simulink model "TTypeInverter_R2022a"  (R2022a)
settings: Solver=ode23t  StartTime=0.0  StopTime=0.2  RelTol=1e-3  EnableMultiTasking=on
values from neighbouring files (symbols this model uses):
  C_c = 30*10^-6    (= 3e-05)    [TTypeInverterVals.m]
  den = abs(G_pr_r_z.Denominator{1,1})    [TTypeInverterVals.m]
  den15 = abs(G_pr_r_15_z.Denominator{1,1})    [TTypeInverterVals.m]
  den21 = abs(G_pr_r_21_z.Denominator{1,1})    [TTypeInverterVals.m]
  den5 = abs(G_pr_r_5_z.Denominator{1,1})    [TTypeInverterVals.m]
  den7 = abs(G_pr_r_7_z.Denominator{1,1})    [TTypeInverterVals.m]
  f_o = 50    [TTypeInverterVals.m]
  G_diff_z = c2d(G_diff_s,Ts,opt)    [ControllerDesign.m]    (also in TTypeInverterVals.m = c2d(G_diff_s,Ts,'foh'))
  Kc = 2.5    [ControllerDesign.m]    (also in TTypeInverterVals.m)
  Klim = 5    [TTypeInverterVals.m]
  Kp = 1/mag/(10^(1.14/20))    [ControllerDesign.m]    (also in TTypeInverterVals.m = 0.9444)
  Kr = omega_c_o/2    (= 3141.59265359)    [ControllerDesign.m]    (also in TTypeInverterVals.m)
  N = 26    [Inductance.m]    (also in TTypeInverterVals.m = [0])
  num = abs(G_pr_r_z.Numerator{1,1})    [TTypeInverterVals.m]
  num15 = abs(G_pr_r_15_z.Numerator{1,1})    [TTypeInverterVals.m]
  num21 = abs(G_pr_r_21_z.Numerator{1,1})    [TTypeInverterVals.m]
  num5 = abs(G_pr_r_5_z.Numerator{1,1})    [TTypeInverterVals.m]
  num7 = abs(G_pr_r_7_z.Numerator{1,1})    [TTypeInverterVals.m]
  omega_o = fo*2*pi    (= 314.159265359)    [ControllerDesign.m]    (also in TTypeInverterVals.m)
  omega_w = 0.1*2*pi    (= 0.628318530718)    [ControllerDesign.m]    (also in TTypeInverterVals.m)
  pr_sat_val = ceil(3*io_nom)    [TTypeInverterVals.m]
  Q = eye(3)    [TTypeInverterVals.m]
  R = [R_iL 0 ... (first row only)    [TTypeInverterVals.m]
  R_l_20p = Vout^2/P_lin_20p    (= 10.58)    [TTypeInverterVals.m]
  R_l_3p = Vout/(P_max_3p/(Vout*3))    (= 2.116)    [TTypeInverterVals.m]
  R_l_80p = Vout^2/P_lin_80p    (= 2.645)    [TTypeInverterVals.m]
  R_l_nl = Vout^2/P_lin    (= 3.11176470588)    [TTypeInverterVals.m]
  R_l_nl_3p = Vout_3p^2/P_lin_3p    [TTypeInverterVals.m]
  R_Lc = 5.6e-3    (= 0.0056)    [TTypeInverterVals.m]
  R_nl_load = Uc^2/(0.66*S_tot)    (= 14.9121893939)    [TTypeInverterVals.m]
  R_nl_load_3p = Uc_3p^2/(0.66*S_tot_3p)    (= 4.97072979798)    [TTypeInverterVals.m]
  R_nl_s = 0.04*Vout^2/S_tot    (= 0.2645)    [TTypeInverterVals.m]
  R_nl_s_3p = 0.04*Vout_3p^2/S_tot_3p    [TTypeInverterVals.m]
  T_sw = 1/f_sw    (= 4.16666666667e-05)    [TTypeInverterVals.m]
  Tcomp = Ts/4    (= 2.60400009204e-06)    [TTypeInverterVals.m]
  Ts = 1/fs    (= 1.04166666667e-05)    [ControllerDesign.m]    (also in KalmanFilter.m = 2.08333333333e-05; TTypeInverterVals.m = 1.04160003681e-05)
  VDC = 800    [TTypeInverterVals.m]
  Vout_amp = Vout*sqrt(2)    [TTypeInverterVals.m]
undefined symbols (not defined in the file or in its folder): a0, a1, b0, b1, Discrete, G_ll_z, Ki, Kpc, KT, kv, Time, UKF_data
libraries: ee_lib x94, nesl_utility x48, fl_lib x39, dspstat3 x15, spsTriangleGeneratorLib x6, ctrlSharedLib x3, spsRMSLib x3, spsTHDLib x3
(part 4 of 5)

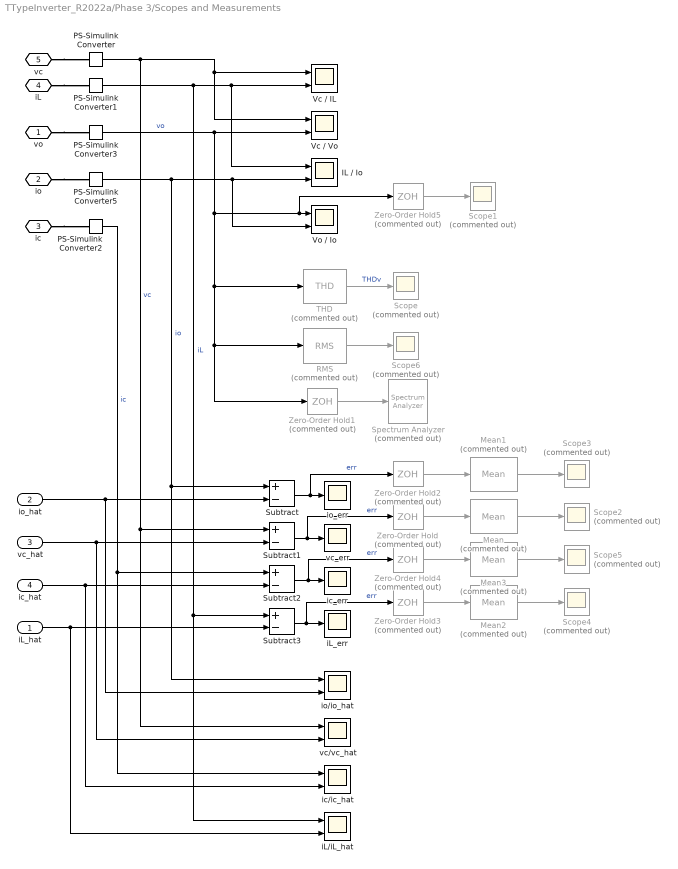
== system TTypeInverter_R2022a/Phase 3/Scopes and Measurements ==
  iL_hat : Inport
  io_hat : Inport  Port=2
  vc_hat : Inport  Port=3
  ic_hat : Inport  Port=4
  IL / Io : Scope  NumInputPorts=2
  Mean{,1..3} (4 alike) : dspstat3/Mean  Commented=on  run=on  InputProcessing=Columns as channels (frame based)  reset_popup=None  directionMode=Each column  dimension=1  roiEnable=off  roiType=Rectangles  roiPortion=Entire ROI  roiOutput=Individual statistics for each ROI  roiFlag=off  roundingMode=Floor  overflowMode=off  outputDataTypeStr=Inherit: Same as accumulator  outputMin=[]  outputMax=[]  outputLastDataTypeStr=Inherit: Same as accumulator
  PS-Simulink Converter{,1..3,5} (5 alike) : nesl_utility/PS-Simulink Converter  PhysicalDomain=network_engine_domain  SubClassName=ps_output  LeftPortType=input  RightPortType=output  PseudoPeriodic=off  Frequencies=[]  VectorFormat=inherit  Unit=inherit  AffineConversion=off
      settings: SourceProductBaseCode=SS,PW,VE
  RMS : spsRMSLib/RMS  Commented=on  TrueRMS=on  Freq=100  RMSInit=230  Ts=0
  Scope{,1..6} (7 alike) : Scope  Commented=on
  Spectrum Analyzer : SpectrumAnalyzer  Commented=on
  Subtract{,1..3} (4 alike) : Sum  Inputs=+-
  THD : spsTHDLib/THD  Commented=on  Freq=50  Ts=0
      settings: SourceProductBaseCode=PS
  Vc / IL : Scope  NumInputPorts=2
  Vc / Vo : Scope  NumInputPorts=2
  Vo / Io : Scope  NumInputPorts=2
  Zero-Order Hold{,2..4} (4 alike) : ZeroOrderHold  Commented=on  SampleTime=Ts/10
  Zero-Order Hold1 : ZeroOrderHold  Commented=on  SampleTime=1/100000
  Zero-Order Hold5 : ZeroOrderHold  Commented=on  SampleTime=T_sw/500
  iL/iL_hat : Scope  NumInputPorts=2
  iL_err : Scope
  ic/ic_hat : Scope  NumInputPorts=2
  ic_err : Scope
  io/io_hat : Scope  NumInputPorts=2
  io_err : Scope
  vc/vc_hat : Scope  NumInputPorts=2
  vc_err : Scope
  vo : PMIOPort  Side=Left
  io : PMIOPort  Port=2  Side=Left
  ic : PMIOPort  Port=3  Side=Left
  iL : PMIOPort  Port=4  Side=Left
  vc : PMIOPort  Port=5  Side=Left
  wires:
  PS-Simulink Converter1/1 -> iL/iL_hat/1, Subtract3/1, IL / Io/1, Vc / IL/2  "iL"
  PS-Simulink Converter/1 -> vc/vc_hat/1, Subtract1/1, Vc / Vo/1, Vc / IL/1  "vc"
  THD/1 -> Scope/1  "THDv"
  PS-Simulink Converter5/1 -> io/io_hat/1, Subtract/1, Vo / Io/2, IL / Io/2  "io"
  Zero-Order Hold1/1 -> Spectrum Analyzer/1
  io_hat/1 -> io/io_hat/2, Subtract/2
  Subtract/1 -> Zero-Order Hold2/1, io_err/1  "err"
  ic_hat/1 -> ic/ic_hat/2, Subtract2/2
  vc_hat/1 -> vc/vc_hat/2, Subtract1/2
  Subtract1/1 -> Zero-Order Hold/1, vc_err/1  "err"
  PS-Simulink Converter2/1 -> ic/ic_hat/1, Subtract2/1  "ic"
  Subtract2/1 -> Zero-Order Hold4/1, ic_err/1  "err"
  Mean/1 -> Scope2/1
  Zero-Order Hold/1 -> Mean/1
  Mean1/1 -> Scope3/1
  Zero-Order Hold2/1 -> Mean1/1
  iL_hat/1 -> iL/iL_hat/2, Subtract3/2
  Subtract3/1 -> Zero-Order Hold3/1, iL_err/1  "err"
  Mean2/1 -> Scope4/1
  Zero-Order Hold3/1 -> Mean2/1
  Mean3/1 -> Scope5/1
  Zero-Order Hold4/1 -> Mean3/1
  RMS/1 -> Scope6/1
  PS-Simulink Converter3/1 -> Vc / Vo/2, Zero-Order Hold5/1, Vo / Io/1, THD/1, RMS/1, Zero-Order Hold1/1  "vo"
  Zero-Order Hold5/1 -> Scope1/1
  connections:
  vc/RConn1 -- PS-Simulink Converter/LConn1
  iL/RConn1 -- PS-Simulink Converter1/LConn1
  vo/RConn1 -- PS-Simulink Converter3/LConn1
  io/RConn1 -- PS-Simulink Converter5/LConn1
  ic/RConn1 -- PS-Simulink Converter2/LConn1

== system TTypeInverter_R2022a/Phase 1/Controllers/Current Controller ==
  iL : Inport
  In : Inport  Port=2
  Add : Sum  Inputs=+++++
  Gain : Gain  Commented=on  Gain=kv
  Impulse Invariant PR - HC15 : Subsystem
  Impulse Invariant PR - HC21 : Subsystem
  Impulse Invariant PR - HC5 : Subsystem
  Impulse Invariant PR - HC7 : Subsystem
  Lead-Lag : Subsystem  Commented=on
  Lead-Lag Net : DiscreteTransferFcn  Commented=on  Numerator=G_ll_z.Numerator{1,1}  Denominator=G_ll_z.Denominator{1,1}  SampleTime=Ts
  P Controller : Gain  Gain=Kc
  PI Controller : Subsystem  Commented=on
  Variable Gain : MATLAB Function  TreatAsAtomicUnit=on
  Out : Outport
  wires:
  Impulse Invariant PR - HC5/1(Out) -> Add/2
  Impulse Invariant PR - HC7/1(Out) -> Add/3
  Gain/1 -> Lead-Lag Net/1
  iL/1 -> Variable Gain/1(iL)
  Add/1 -> Out/1
  P Controller/1 -> Add/1
  In/1 -> Variable Gain/2(e_in)
  Variable Gain/1(e_out) -> P Controller/1, Impulse Invariant PR - HC21/1(e_out), Impulse Invariant PR - HC15/1(e_out), Impulse Invariant PR - HC7/1(In), Impulse Invariant PR - HC5/1(In)
  Impulse Invariant PR - HC15/1(Out) -> Add/4
  Impulse Invariant PR - HC21/1(Out) -> Add/5

== system TTypeInverter_R2022a/Phase 1/Controllers/Voltage Controller ==
  note: Pre-warped Tustin PR with HC
  In : Inport
  Add : Sum
  Fifth Harmonic : Subsystem  Commented=on
  Fundamental : Subsystem  Commented=on
  Impulse Invariant PR - Fundamental : Subsystem
  Multiply2 : Gain  Gain=Kp
  Non-prewarped Tustin-based PR : Subsystem  Commented=on
  Saturation : Saturate  UpperLimit=pr_sat_val  LowerLimit=-pr_sat_val
  Seventh Harmonic : Subsystem  Commented=on
  Sum1 : Sum  Inputs=-|+
  Third Harmonic : Subsystem  Commented=on
  Out : Outport
  wires:
  Multiply2/1 -> Add/1
  Saturation/1 -> Out/1, Sum1/1
  Add/1 -> Saturation/1, Sum1/2
  Impulse Invariant PR - Fundamental/1(Out) -> Add/2
  Sum1/1 -> Impulse Invariant PR - Fundamental/2(Anti-Windup)
  In/1 -> Impulse Invariant PR - Fundamental/1(e_out), Multiply2/1

== system TTypeInverter_R2022a/Phase 1/Kalman Filter - Unscented/Unscented Kalman Filter ==
  u : Inport
  y : Inport  Port=2
  Constant : Constant  Value=UKF_data.x_0_l1  VectorParams1D=off
  Constant1 : Constant  Value=UKF_data.P_0  VectorParams1D=off
  Constant4 : Constant  Value=UKF_data.y_0_l1  VectorParams1D=off
  Delay : Delay  DelayLength=1  InitialConditionSource=Input port  SampleTime=Ts
      settings: InputPortMap=u0,p4
  Delay1 : Delay  DelayLength=1  InitialConditionSource=Input port  SampleTime=Ts
      settings: InputPortMap=u0,p4
  Delay4 : Delay  DelayLength=1  InitialConditionSource=Input port  SampleTime=Ts
      settings: InputPortMap=u0,p4
  Demux : Demux  Outputs=2
  Demux1 : Demux  Outputs=3
  Predict Step : MATLAB Function  TreatAsAtomicUnit=on  mask{UKF_struct=UKF_data}
      mask prompts: UKF_struct "Data Structure"
  Scope : Scope  NumInputPorts=2
  Scope1 : Scope  NumInputPorts=3
  Update Step : MATLAB Function  TreatAsAtomicUnit=on  mask{UKF_struct=UKF_data}
      mask prompts: UKF_struct "Data Structure"
  xhat : Outport
  yhat : Outport  Port=2
  wires:
  Constant/1 -> Delay/2
  Constant1/1 -> Delay1/2
  Update Step/1(yhat) -> yhat/1
  Delay1/1 -> Update Step/3(P_minus)
  u/1 -> Predict Step/3(u_k)
  Predict Step/3(xhat_minus) -> Demux1/1, Delay/1
  Predict Step/2(P_minus) -> Delay1/1
  Delay/1 -> Update Step/4(xhat_minus)
  Constant4/1 -> Delay4/2
  Predict Step/1(yhat_minus) -> Delay4/1, Demux/1
  Delay4/1 -> Update Step/2(yhat_minus)
  y/1 -> Update Step/1(y)
  Demux/1 -> Scope/1  "iL"
  Demux/2 -> Scope/2  "vc"
  Demux1/1 -> Scope1/1  "iL"
  Demux1/2 -> Scope1/2  "vcap"
  Demux1/3 -> Scope1/3  "ic"
  Update Step/2(xhat) -> Predict Step/1(xhat_k), xhat/1
  Update Step/3(P) -> Predict Step/2(P_k)

== system TTypeInverter_R2022a/Phase 2/Controllers/Current Controller ==
  iL : Inport
  In : Inport  Port=2
  Add : Sum  Inputs=+++++
  Gain : Gain  Commented=on  Gain=kv
  Impulse Invariant PR - HC15 : Subsystem
  Impulse Invariant PR - HC21 : Subsystem
  Impulse Invariant PR - HC5 : Subsystem
  Impulse Invariant PR - HC7 : Subsystem
  Lead-Lag : Subsystem  Commented=on
  Lead-Lag Net : DiscreteTransferFcn  Commented=on  Numerator=G_ll_z.Numerator{1,1}  Denominator=G_ll_z.Denominator{1,1}  SampleTime=Ts
  P Controller : Gain  Gain=Kc
  PI Controller : Subsystem  Commented=on
  Variable Gain : MATLAB Function  TreatAsAtomicUnit=on
  Out : Outport
  wires:
  Impulse Invariant PR - HC5/1(Out) -> Add/2
  Impulse Invariant PR - HC7/1(Out) -> Add/3
  Gain/1 -> Lead-Lag Net/1
  iL/1 -> Variable Gain/1(iL)
  Add/1 -> Out/1
  P Controller/1 -> Add/1
  In/1 -> Variable Gain/2(e_in)
  Variable Gain/1(e_out) -> P Controller/1, Impulse Invariant PR - HC21/1(e_out), Impulse Invariant PR - HC15/1(e_out), Impulse Invariant PR - HC7/1(In), Impulse Invariant PR - HC5/1(In)
  Impulse Invariant PR - HC15/1(Out) -> Add/4
  Impulse Invariant PR - HC21/1(Out) -> Add/5

== system TTypeInverter_R2022a/Phase 2/Controllers/Voltage Controller ==
  note: Pre-warped Tustin PR with HC
  In : Inport
  Add : Sum
  Fifth Harmonic : Subsystem  Commented=on
  Fundamental : Subsystem  Commented=on
  Impulse Invariant PR - Fundamental : Subsystem
  Multiply2 : Gain  Gain=Kp
  Non-prewarped Tustin-based PR : Subsystem  Commented=on
  Saturation : Saturate  UpperLimit=pr_sat_val  LowerLimit=-pr_sat_val
  Seventh Harmonic : Subsystem  Commented=on
  Sum1 : Sum  Inputs=-|+
  Third Harmonic : Subsystem  Commented=on
  Out : Outport
  wires:
  Multiply2/1 -> Add/1
  Saturation/1 -> Out/1, Sum1/1
  Add/1 -> Saturation/1, Sum1/2
  Impulse Invariant PR - Fundamental/1(Out) -> Add/2
  Sum1/1 -> Impulse Invariant PR - Fundamental/2(Anti-Windup)
  In/1 -> Impulse Invariant PR - Fundamental/1(e_out), Multiply2/1

== system TTypeInverter_R2022a/Phase 2/Kalman Filter - Unscented/Unscented Kalman Filter ==
  u : Inport
  y : Inport  Port=2
  Constant : Constant  Value=UKF_data.x_0_l2  VectorParams1D=off
  Constant1 : Constant  Value=UKF_data.P_0  VectorParams1D=off
  Constant4 : Constant  Value=UKF_data.y_0_l2  VectorParams1D=off
  Delay : Delay  DelayLength=1  InitialConditionSource=Input port  SampleTime=Ts
      settings: InputPortMap=u0,p4
  Delay1 : Delay  DelayLength=1  InitialConditionSource=Input port  SampleTime=Ts
      settings: InputPortMap=u0,p4
  Delay4 : Delay  DelayLength=1  InitialConditionSource=Input port  SampleTime=Ts
      settings: InputPortMap=u0,p4
  Demux : Demux  Outputs=2
  Demux1 : Demux  Outputs=3
  Predict Step : MATLAB Function  TreatAsAtomicUnit=on  mask{UKF_struct=UKF_data}
      mask prompts: UKF_struct "Data Structure"
  Scope : Scope  NumInputPorts=2
  Scope1 : Scope  NumInputPorts=3
  Update Step : MATLAB Function  TreatAsAtomicUnit=on  mask{UKF_struct=UKF_data}
      mask prompts: UKF_struct "Data Structure"
  xhat : Outport
  yhat : Outport  Port=2
  wires:
  Constant/1 -> Delay/2
  Constant1/1 -> Delay1/2
  Update Step/1(yhat) -> yhat/1
  Delay1/1 -> Update Step/3(P_minus)
  u/1 -> Predict Step/3(u_k)
  Predict Step/3(xhat_minus) -> Demux1/1, Delay/1
  Predict Step/2(P_minus) -> Delay1/1
  Delay/1 -> Update Step/4(xhat_minus)
  Constant4/1 -> Delay4/2
  Predict Step/1(yhat_minus) -> Delay4/1, Demux/1
  Delay4/1 -> Update Step/2(yhat_minus)
  y/1 -> Update Step/1(y)
  Demux/1 -> Scope/1  "iL"
  Demux/2 -> Scope/2  "vc"
  Demux1/1 -> Scope1/1  "iL"
  Demux1/2 -> Scope1/2  "vcap"
  Demux1/3 -> Scope1/3  "ic"
  Update Step/2(xhat) -> Predict Step/1(xhat_k), xhat/1
  Update Step/3(P) -> Predict Step/2(P_k)

== system TTypeInverter_R2022a/Phase 3/Controllers/Current Controller ==
  iL : Inport
  In : Inport  Port=2
  Add : Sum  Inputs=+++++
  Gain : Gain  Commented=on  Gain=kv
  Impulse Invariant PR - HC15 : Subsystem
  Impulse Invariant PR - HC21 : Subsystem
  Impulse Invariant PR - HC5 : Subsystem
  Impulse Invariant PR - HC7 : Subsystem
  Lead-Lag : Subsystem  Commented=on
  Lead-Lag Net : DiscreteTransferFcn  Commented=on  Numerator=G_ll_z.Numerator{1,1}  Denominator=G_ll_z.Denominator{1,1}  SampleTime=Ts
  P Controller : Gain  Gain=Kc
  PI Controller : Subsystem  Commented=on
  Variable Gain : MATLAB Function  TreatAsAtomicUnit=on
  Out : Outport
  wires:
  Impulse Invariant PR - HC5/1(Out) -> Add/2
  Impulse Invariant PR - HC7/1(Out) -> Add/3
  Gain/1 -> Lead-Lag Net/1
  iL/1 -> Variable Gain/1(iL)
  Add/1 -> Out/1
  P Controller/1 -> Add/1
  In/1 -> Variable Gain/2(e_in)
  Variable Gain/1(e_out) -> P Controller/1, Impulse Invariant PR - HC21/1(e_out), Impulse Invariant PR - HC15/1(e_out), Impulse Invariant PR - HC7/1(In), Impulse Invariant PR - HC5/1(In)
  Impulse Invariant PR - HC15/1(Out) -> Add/4
  Impulse Invariant PR - HC21/1(Out) -> Add/5

== system TTypeInverter_R2022a/Phase 3/Controllers/Voltage Controller ==
  note: Pre-warped Tustin PR with HC
  In : Inport
  Add : Sum
  Fifth Harmonic : Subsystem  Commented=on
  Fundamental : Subsystem  Commented=on
  Impulse Invariant PR - Fundamental : Subsystem
  Multiply2 : Gain  Gain=Kp
  Non-prewarped Tustin-based PR : Subsystem  Commented=on
  Saturation : Saturate  UpperLimit=pr_sat_val  LowerLimit=-pr_sat_val
  Seventh Harmonic : Subsystem  Commented=on
  Sum1 : Sum  Inputs=-|+
  Third Harmonic : Subsystem  Commented=on
  Out : Outport
  wires:
  Multiply2/1 -> Add/1
  Saturation/1 -> Out/1, Sum1/1
  Add/1 -> Saturation/1, Sum1/2
  Impulse Invariant PR - Fundamental/1(Out) -> Add/2
  Sum1/1 -> Impulse Invariant PR - Fundamental/2(Anti-Windup)
  In/1 -> Impulse Invariant PR - Fundamental/1(e_out), Multiply2/1

== system TTypeInverter_R2022a/Phase 3/Kalman Filter - Unscented/Unscented Kalman Filter ==
  u : Inport
  y : Inport  Port=2
  Constant : Constant  Value=UKF_data.x_0_l3  VectorParams1D=off
  Constant1 : Constant  Value=UKF_data.P_0  VectorParams1D=off
  Constant4 : Constant  Value=UKF_data.y_0_l3  VectorParams1D=off
  Delay : Delay  DelayLength=1  InitialConditionSource=Input port  SampleTime=Ts
      settings: InputPortMap=u0,p4
  Delay1 : Delay  DelayLength=1  InitialConditionSource=Input port  SampleTime=Ts
      settings: InputPortMap=u0,p4
  Delay4 : Delay  DelayLength=1  InitialConditionSource=Input port  SampleTime=Ts
      settings: InputPortMap=u0,p4
  Demux : Demux  Outputs=2
  Demux1 : Demux  Outputs=3
  Predict Step : MATLAB Function  TreatAsAtomicUnit=on  mask{UKF_struct=UKF_data}
      mask prompts: UKF_struct "Data Structure"
  Scope : Scope  NumInputPorts=2
  Scope1 : Scope  NumInputPorts=3
  Update Step : MATLAB Function  TreatAsAtomicUnit=on  mask{UKF_struct=UKF_data}
      mask prompts: UKF_struct "Data Structure"
  xhat : Outport
  yhat : Outport  Port=2
  wires:
  Constant/1 -> Delay/2
  Constant1/1 -> Delay1/2
  Update Step/1(yhat) -> yhat/1
  Delay1/1 -> Update Step/3(P_minus)
  u/1 -> Predict Step/3(u_k)
  Predict Step/3(xhat_minus) -> Demux1/1, Delay/1
  Predict Step/2(P_minus) -> Delay1/1
  Delay/1 -> Update Step/4(xhat_minus)
  Constant4/1 -> Delay4/2
  Predict Step/1(yhat_minus) -> Delay4/1, Demux/1
  Delay4/1 -> Update Step/2(yhat_minus)
  y/1 -> Update Step/1(y)
  Demux/1 -> Scope/1  "iL"
  Demux/2 -> Scope/2  "vc"
  Demux1/1 -> Scope1/1  "iL"
  Demux1/2 -> Scope1/2  "vcap"
  Demux1/3 -> Scope1/3  "ic"
  Update Step/2(xhat) -> Predict Step/1(xhat_k), xhat/1
  Update Step/3(P) -> Predict Step/2(P_k)

== system TTypeInverter_R2022a/Phase 1/Controllers/Current Controller/Impulse Invariant PR - HC15 ==
  e_out : Inport
  Anti-Windup : Inport  Port=2
  1/b0 : Gain  Gain=1/den15(1)
  Delay{1,3..5} (4 alike) : Delay  DelayLength=1  SampleTime=Ts
  Klim : Gain  Gain=Klim
  Sum : Sum  Inputs=|+-
  Sum3 : Sum  Inputs=|+-
  Sum4 : Sum  Inputs=|++
  Sum5 : Sum  Inputs=+-|
  a0 : Gain  Gain=num15(1)
  a1 : Gain  Gain=num15(2)
  b1 : Gain  Gain=den15(2)
  b2 : Gain  Gain=den15(3)
  Out : Outport
  wires:
  Delay3/1 -> a1/1  "e(n-1)"
  Delay5/1 -> b2/1  "y(n-2)"
  1/b0/1 -> Out/1, Delay4/1  "y(n)"
  Sum3/1 -> Sum4/1
  Sum4/1 -> 1/b0/1
  b2/1 -> Sum5/2
  Sum5/1 -> Sum4/2
  b1/1 -> Sum5/1
  Delay4/1 -> Delay5/1, b1/1  "y(n-1)"
  a0/1 -> Sum3/1
  a1/1 -> Sum3/2
  Klim/1 -> Sum/2
  Anti-Windup/1 -> Delay1/1
  Delay1/1 -> Klim/1
  Sum/1 -> a0/1, Delay3/1  "e(n)"
  e_out/1 -> Sum/1

== system TTypeInverter_R2022a/Phase 1/Controllers/Current Controller/Impulse Invariant PR - HC21 ==
  e_out : Inport
  Anti-Windup : Inport  Port=2
  1/b0 : Gain  Gain=1/den21(1)
  Delay{1,3..5} (4 alike) : Delay  DelayLength=1  SampleTime=Ts
  Klim : Gain  Gain=Klim
  Sum : Sum  Inputs=|+-
  Sum3 : Sum  Inputs=|+-
  Sum4 : Sum  Inputs=|++
  Sum5 : Sum  Inputs=+-|
  a0 : Gain  Gain=num21(1)
  a1 : Gain  Gain=num21(2)
  b1 : Gain  Gain=den21(2)
  b2 : Gain  Gain=den21(3)
  Out : Outport
  wires:
  Delay3/1 -> a1/1  "e(n-1)"
  Delay5/1 -> b2/1  "y(n-2)"
  1/b0/1 -> Out/1, Delay4/1  "y(n)"
  Sum3/1 -> Sum4/1
  Sum4/1 -> 1/b0/1
  b2/1 -> Sum5/2
  Sum5/1 -> Sum4/2
  b1/1 -> Sum5/1
  Delay4/1 -> Delay5/1, b1/1  "y(n-1)"
  a0/1 -> Sum3/1
  a1/1 -> Sum3/2
  Klim/1 -> Sum/2
  Anti-Windup/1 -> Delay1/1
  Delay1/1 -> Klim/1
  Sum/1 -> a0/1, Delay3/1  "e(n)"
  e_out/1 -> Sum/1

== system TTypeInverter_R2022a/Phase 1/Controllers/Current Controller/Impulse Invariant PR - HC5 ==
  In : Inport
  Anti-Windup : Inport  Port=2
  1/b0 : Gain  Gain=1/den5(1)
  Delay{1,3..5} (4 alike) : Delay  DelayLength=1  SampleTime=Ts
  Klim : Gain  Gain=Klim
  Sum : Sum  Inputs=|+-
  Sum3 : Sum  Inputs=|+-
  Sum4 : Sum  Inputs=|++
  Sum5 : Sum  Inputs=+-|
  a0 : Gain  Gain=num5(1)
  a1 : Gain  Gain=num5(2)
  b1 : Gain  Gain=den5(2)
  b2 : Gain  Gain=den5(3)
  Out : Outport
  wires:
  Delay3/1 -> a1/1  "e(n-1)"
  Delay5/1 -> b2/1  "y(n-2)"
  1/b0/1 -> Out/1, Delay4/1  "y(n)"
  Sum3/1 -> Sum4/1
  Sum4/1 -> 1/b0/1
  b2/1 -> Sum5/2
  Sum5/1 -> Sum4/2
  b1/1 -> Sum5/1
  Delay4/1 -> Delay5/1, b1/1  "y(n-1)"
  a0/1 -> Sum3/1
  a1/1 -> Sum3/2
  Delay1/1 -> Klim/1
  Klim/1 -> Sum/2
  Anti-Windup/1 -> Delay1/1
  Sum/1 -> a0/1, Delay3/1  "e(n)"
  In/1 -> Sum/1

== system TTypeInverter_R2022a/Phase 1/Controllers/Current Controller/Impulse Invariant PR - HC7 ==
  In : Inport
  Anti-Windup : Inport  Port=2
  1/b0 : Gain  Gain=1/den7(1)
  Delay{1,3..5} (4 alike) : Delay  DelayLength=1  SampleTime=Ts
  Klim : Gain  Gain=Klim
  Sum : Sum  Inputs=|+-
  Sum3 : Sum  Inputs=|+-
  Sum4 : Sum  Inputs=|++
  Sum5 : Sum  Inputs=+-|
  a0 : Gain  Gain=num7(1)
  a1 : Gain  Gain=num7(2)
  b1 : Gain  Gain=den7(2)
  b2 : Gain  Gain=den7(3)
  Out : Outport
  wires:
  Delay3/1 -> a1/1  "e(n-1)"
  Delay5/1 -> b2/1  "y(n-2)"
  1/b0/1 -> Out/1, Delay4/1  "y(n)"
  Sum3/1 -> Sum4/1
  Sum4/1 -> 1/b0/1
  b2/1 -> Sum5/2
  Sum5/1 -> Sum4/2
  b1/1 -> Sum5/1
  Delay4/1 -> Delay5/1, b1/1  "y(n-1)"
  a0/1 -> Sum3/1
  a1/1 -> Sum3/2
  Klim/1 -> Sum/2
  Anti-Windup/1 -> Delay1/1
  Delay1/1 -> Klim/1
  Sum/1 -> a0/1, Delay3/1  "e(n)"
  In/1 -> Sum/1

== system TTypeInverter_R2022a/Phase 1/Controllers/Current Controller/Lead-Lag ==
  In : Inport
  Delay : Delay  DelayLength=1  SampleTime=Ts
  Delay1 : Delay  DelayLength=1  SampleTime=Ts
  Gain : Gain  Gain=C_c
  Gain1 : Gain
  Sum : Sum  Inputs=|++
  Sum1 : Sum  Inputs=|++
  a0 : Gain  Gain=a0
  a1 : Gain  Gain=a1
  b0 : Gain  Gain=b0
  b1 : Gain  Gain=b1
  Out : Outport
  wires:
  Gain1/1 -> Out/1
  Gain/1 -> Gain1/1
  In/1 -> Delay/1, a0/1  "e(n)"
  a0/1 -> Sum/1
  Delay/1 -> a1/1  "e(n-1)"
  a1/1 -> Sum/2
  Sum/1 -> Sum1/1
  Delay1/1 -> b1/1  "y(n-1)"
  b1/1 -> Sum1/2
  Sum1/1 -> b0/1
  b0/1 -> Delay1/1, Gain/1  "y(n)"

== system TTypeInverter_R2022a/Phase 1/Controllers/Current Controller/PI Controller ==
  In : Inport
  Delay : Delay  DelayLength=1  SampleTime=Ts
  Gain1 : Gain  Gain=Kpc
  Gain2 : Gain  Gain=Ki
  Gain3 : Gain  Gain=Ts
  Sum2 : Sum  Inputs=++|
  Sum3 : Sum  Inputs=|++
  Out : Outport
  wires:
  Gain1/1 -> Sum2/1
  Gain2/1 -> Gain3/1
  Sum3/1 -> Sum2/2, Delay/1
  Gain3/1 -> Sum3/1
  Delay/1 -> Sum3/2
  In/1 -> Gain1/1, Gain2/1
  Sum2/1 -> Out/1

== system TTypeInverter_R2022a/Phase 1/Controllers/Voltage Controller/Fifth Harmonic ==
  In : Inport
  Anti-Windup : Inport  Port=2
  1/b0 : Gain  Gain=1/(KT(3)*KT(3)+2*omega_w(3)*KT(3)+5*5*omega_o*omega_o)
  Delay1 : Delay  DelayLength=1  SampleTime=Ts
  Delay3 : Delay  SampleTime=Ts
  Delay4 : Delay  DelayLength=1  SampleTime=Ts
  Delay5 : Delay  DelayLength=1  SampleTime=Ts
  Klim : Gain  Gain=Klim
  Sum : Sum  Inputs=|+-
  Sum3 : Sum  Inputs=|+-
  Sum4 : Sum  Inputs=|++
  Sum5 : Sum  Inputs=+-|
  a1 : Gain  Gain=2*Kr(3)*KT(3)*omega_w(3)
  b1 : Gain  Gain=2*KT(3)*KT(3)-2*5*5*omega_o*omega_o
  b2 : Gain  Gain=KT(3)*KT(3)+2*omega_w(3)*KT(3)-5*5*omega_o*omega_o
  Out : Outport
  wires:
  Delay3/1 -> Sum3/2  "e(n-2)"
  Delay5/1 -> b2/1  "y(n-2)"
  Klim/1 -> Sum/2
  1/b0/1 -> Out/1, Delay4/1  "y(n)"
  a1/1 -> Sum4/1
  Sum4/1 -> 1/b0/1
  Sum3/1 -> a1/1
  b2/1 -> Sum5/2
  Sum5/1 -> Sum4/2
  Sum/1 -> Sum3/1, Delay3/1  "e(n)"
  b1/1 -> Sum5/1
  Delay4/1 -> Delay5/1, b1/1  "y(n-1)"
  In/1 -> Sum/1
  Delay1/1 -> Klim/1
  Anti-Windup/1 -> Delay1/1

== system TTypeInverter_R2022a/Phase 1/Controllers/Voltage Controller/Fundamental ==
  In : Inport
  Anti-Windup : Inport  Port=2
  1/b0 : Gain  Gain=1/(KT(1)*KT(1)+2*omega_w(1)*KT(1)+omega_o*omega_o)
  Delay1 : Delay  DelayLength=1  SampleTime=Ts
  Delay3 : Delay  SampleTime=Ts
  Delay4 : Delay  DelayLength=1  SampleTime=Ts
  Delay5 : Delay  DelayLength=1  SampleTime=Ts
  Klim : Gain  Gain=Klim
  Sum : Sum  Inputs=|+-
  Sum3 : Sum  Inputs=|+-
  Sum4 : Sum  Inputs=|++
  Sum5 : Sum  Inputs=+-|
  a1 : Gain  Gain=2*Kr(1)*KT(1)*omega_w(1)
  b1 : Gain  Gain=2*KT(1)*KT(1)-2*omega_o*omega_o
  b2 : Gain  Gain=KT(1)*KT(1)+2*omega_w(1)*KT(1)-omega_o*omega_o
  Out : Outport
  wires:
  Delay3/1 -> Sum3/2  "e(n-2)"
  Delay5/1 -> b2/1  "y(n-2)"
  Klim/1 -> Sum/2
  1/b0/1 -> Out/1, Delay4/1  "y(n)"
  a1/1 -> Sum4/1
  Sum4/1 -> 1/b0/1
  Sum3/1 -> a1/1
  b2/1 -> Sum5/2
  Sum5/1 -> Sum4/2
  Sum/1 -> Sum3/1, Delay3/1  "e(n)"
  b1/1 -> Sum5/1
  Delay4/1 -> Delay5/1, b1/1  "y(n-1)"
  In/1 -> Sum/1
  Delay1/1 -> Klim/1
  Anti-Windup/1 -> Delay1/1

== system TTypeInverter_R2022a/Phase 1/Controllers/Voltage Controller/Impulse Invariant PR - Fundamental ==
  e_out : Inport
  Anti-Windup : Inport  Port=2
  1/b0 : Gain  Gain=1/den(1)
  Delay{1,3..5} (4 alike) : Delay  DelayLength=1  SampleTime=Ts
  Klim : Gain  Gain=Klim
  Sum : Sum  Inputs=|+-
  Sum3 : Sum  Inputs=|+-
  Sum4 : Sum  Inputs=|++
  Sum5 : Sum  Inputs=+-|
  a0 : Gain  Gain=num(1)
  a1 : Gain  Gain=num(2)
  b1 : Gain  Gain=den(2)
  b2 : Gain  Gain=den(3)
  Out : Outport
  wires:
  Delay3/1 -> a1/1  "e(n-1)"
  Delay5/1 -> b2/1  "y(n-2)"
  Klim/1 -> Sum/2
  1/b0/1 -> Out/1, Delay4/1  "y(n)"
  Sum3/1 -> Sum4/1
  Sum4/1 -> 1/b0/1
  b2/1 -> Sum5/2
  Sum5/1 -> Sum4/2
  Sum/1 -> a0/1, Delay3/1  "e(n)"
  b1/1 -> Sum5/1
  Delay4/1 -> Delay5/1, b1/1  "y(n-1)"
  e_out/1 -> Sum/1
  Delay1/1 -> Klim/1
  Anti-Windup/1 -> Delay1/1
  a0/1 -> Sum3/1
  a1/1 -> Sum3/2

== system TTypeInverter_R2022a/Phase 1/Controllers/Voltage Controller/Non-prewarped Tustin-based PR ==
  In1 : Inport
  1/(Ts*Ts*omega_0*omega_0+4*Ts*omega_w+4) : Gain  Gain=1/(Ts*Ts*omega_o*omega_o+4*Ts*omega_w(1)+4)
  2*Ts*Ts*omega_0*omega_0 : Gain  Gain=2*Ts*Ts*omega_o*omega_o-8
  4*Ts*omega_w : Gain  Gain=4*Ts*omega_w(1)
  4*Ts*omega_w! : Gain  Gain=4*Ts*omega_w(1)
  Add1 : Sum
  Delay3 : Delay  SampleTime=Ts
  Delay4 : Delay  DelayLength=1  SampleTime=Ts
  Delay5 : Delay  DelayLength=1  SampleTime=Ts
  Multiply2 : Gain  Gain=Kp
  Multiply3 : Gain  Gain=Kr(1)
  Saturation : Saturate  UpperLimit=pr_sat_val  LowerLimit=-pr_sat_val
  Sum3 : Sum  Inputs=|+-
  Sum4 : Sum  Inputs=|+-
  Sum5 : Sum  Inputs=++|
  Ts*Ts*omega_0*omega_0-4*Ts*omega_w : Gain  Gain=Ts*Ts*omega_o*omega_o-4*Ts*omega_w(1)+4
  Out1 : Outport
  wires:
  Multiply2/1 -> Add1/1
  Delay4/1 -> Delay5/1, 2*Ts*Ts*omega_0*omega_0/1
  Delay5/1 -> Ts*Ts*omega_0*omega_0-4*Ts*omega_w/1
  Multiply3/1 -> Delay3/1, 4*Ts*omega_w/1
  Delay3/1 -> 4*Ts*omega_w!/1
  Sum3/1 -> Sum4/1
  In1/1 -> Multiply3/1, Multiply2/1
  4*Ts*omega_w/1 -> Sum3/1
  Saturation/1 -> Out1/1
  Ts*Ts*omega_0*omega_0-4*Ts*omega_w/1 -> Sum5/2
  4*Ts*omega_w!/1 -> Sum3/2
  Sum5/1 -> Sum4/2
  Sum4/1 -> 1/(Ts*Ts*omega_0*omega_0+4*Ts*omega_w+4)/1
  Add1/1 -> Saturation/1
  1/(Ts*Ts*omega_0*omega_0+4*Ts*omega_w+4)/1 -> Add1/2, Delay4/1
  2*Ts*Ts*omega_0*omega_0/1 -> Sum5/1

== system TTypeInverter_R2022a/Phase 1/Controllers/Voltage Controller/Seventh Harmonic ==
  In : Inport
  Anti-Windup : Inport  Port=2
  1/b0 : Gain  Gain=1/(KT(4)*KT(4)+2*omega_w(4)*KT(4)+7*omega_o*omega_o)
  Delay1 : Delay  DelayLength=1  SampleTime=Ts
  Delay3 : Delay  SampleTime=Ts
  Delay4 : Delay  DelayLength=1  SampleTime=Ts
  Delay5 : Delay  DelayLength=1  SampleTime=Ts
  Klim : Gain  Gain=Klim
  Sum : Sum  Inputs=|+-
  Sum3 : Sum  Inputs=|+-
  Sum4 : Sum  Inputs=|++
  Sum5 : Sum  Inputs=+-|
  a1 : Gain  Gain=2*Kr(4)*KT(4)*omega_w(4)
  b1 : Gain  Gain=2*KT(4)*KT(4)-2*7*omega_o*omega_o
  b2 : Gain  Gain=KT(4)*KT(4)+2*omega_w(4)*KT(4)-7*omega_o*omega_o
  Out : Outport
  wires:
  Delay3/1 -> Sum3/2  "e(n-2)"
  Delay5/1 -> b2/1  "y(n-2)"
  Klim/1 -> Sum/2
  1/b0/1 -> Out/1, Delay4/1  "y(n)"
  a1/1 -> Sum4/1
  Sum4/1 -> 1/b0/1
  Sum3/1 -> a1/1
  b2/1 -> Sum5/2
  Sum5/1 -> Sum4/2
  Sum/1 -> Sum3/1, Delay3/1  "e(n)"
  b1/1 -> Sum5/1
  Delay4/1 -> Delay5/1, b1/1  "y(n-1)"
  In/1 -> Sum/1
  Delay1/1 -> Klim/1
  Anti-Windup/1 -> Delay1/1

== system TTypeInverter_R2022a/Phase 1/Controllers/Voltage Controller/Third Harmonic ==
  In : Inport
  Anti-Windup : Inport  Port=2
  1/b0 : Gain  Gain=1/(KT(2)*KT(2)+2*omega_w(2)*KT(2)+3*3*omega_o*omega_o)
  Delay1 : Delay  DelayLength=1  SampleTime=Ts
  Delay3 : Delay  SampleTime=Ts
  Delay4 : Delay  DelayLength=1  SampleTime=Ts
  Delay5 : Delay  DelayLength=1  SampleTime=Ts
  Klim : Gain  Gain=Klim
  Sum : Sum  Inputs=|+-
  Sum3 : Sum  Inputs=|+-
  Sum4 : Sum  Inputs=|++
  Sum5 : Sum  Inputs=+-|
  a1 : Gain  Gain=2*Kr(2)*KT(2)*omega_w(2)
  b1 : Gain  Gain=2*KT(2)*KT(2)-2*3*3*omega_o*omega_o
  b2 : Gain  Gain=KT(2)*KT(2)+2*omega_w(2)*KT(2)-3*3*omega_o*omega_o
  Out : Outport
  wires:
  Delay3/1 -> Sum3/2  "e(n-2)"
  Delay5/1 -> b2/1  "y(n-2)"
  Klim/1 -> Sum/2
  1/b0/1 -> Out/1, Delay4/1  "y(n)"
  a1/1 -> Sum4/1
  Sum4/1 -> 1/b0/1
  Sum3/1 -> a1/1
  b2/1 -> Sum5/2
  Sum5/1 -> Sum4/2
  Sum/1 -> Sum3/1, Delay3/1  "e(n)"
  b1/1 -> Sum5/1
  Delay4/1 -> Delay5/1, b1/1  "y(n-1)"
  In/1 -> Sum/1
  Delay1/1 -> Klim/1
  Anti-Windup/1 -> Delay1/1

== system TTypeInverter_R2022a/Phase 2/Controllers/Current Controller/Impulse Invariant PR - HC15 ==
  e_out : Inport
  Anti-Windup : Inport  Port=2
  1/b0 : Gain  Gain=1/den15(1)
  Delay{1,3..5} (4 alike) : Delay  DelayLength=1  SampleTime=Ts
  Klim : Gain  Gain=Klim
  Sum : Sum  Inputs=|+-
  Sum3 : Sum  Inputs=|+-
  Sum4 : Sum  Inputs=|++
  Sum5 : Sum  Inputs=+-|
  a0 : Gain  Gain=num15(1)
  a1 : Gain  Gain=num15(2)
  b1 : Gain  Gain=den15(2)
  b2 : Gain  Gain=den15(3)
  Out : Outport
  wires:
  Delay3/1 -> a1/1  "e(n-1)"
  Delay5/1 -> b2/1  "y(n-2)"
  1/b0/1 -> Out/1, Delay4/1  "y(n)"
  Sum3/1 -> Sum4/1
  Sum4/1 -> 1/b0/1
  b2/1 -> Sum5/2
  Sum5/1 -> Sum4/2
  b1/1 -> Sum5/1
  Delay4/1 -> Delay5/1, b1/1  "y(n-1)"
  a0/1 -> Sum3/1
  a1/1 -> Sum3/2
  Klim/1 -> Sum/2
  Anti-Windup/1 -> Delay1/1
  Delay1/1 -> Klim/1
  Sum/1 -> a0/1, Delay3/1  "e(n)"
  e_out/1 -> Sum/1

== system TTypeInverter_R2022a/Phase 2/Controllers/Current Controller/Impulse Invariant PR - HC21 ==
  e_out : Inport
  Anti-Windup : Inport  Port=2
  1/b0 : Gain  Gain=1/den21(1)
  Delay{1,3..5} (4 alike) : Delay  DelayLength=1  SampleTime=Ts
  Klim : Gain  Gain=Klim
  Sum : Sum  Inputs=|+-
  Sum3 : Sum  Inputs=|+-
  Sum4 : Sum  Inputs=|++
  Sum5 : Sum  Inputs=+-|
  a0 : Gain  Gain=num21(1)
  a1 : Gain  Gain=num21(2)
  b1 : Gain  Gain=den21(2)
  b2 : Gain  Gain=den21(3)
  Out : Outport
  wires:
  Delay3/1 -> a1/1  "e(n-1)"
  Delay5/1 -> b2/1  "y(n-2)"
  1/b0/1 -> Out/1, Delay4/1  "y(n)"
  Sum3/1 -> Sum4/1
  Sum4/1 -> 1/b0/1
  b2/1 -> Sum5/2
  Sum5/1 -> Sum4/2
  b1/1 -> Sum5/1
  Delay4/1 -> Delay5/1, b1/1  "y(n-1)"
  a0/1 -> Sum3/1
  a1/1 -> Sum3/2
  Klim/1 -> Sum/2
  Anti-Windup/1 -> Delay1/1
  Delay1/1 -> Klim/1
  Sum/1 -> a0/1, Delay3/1  "e(n)"
  e_out/1 -> Sum/1

== system TTypeInverter_R2022a/Phase 2/Controllers/Current Controller/Impulse Invariant PR - HC5 ==
  In : Inport
  Anti-Windup : Inport  Port=2
  1/b0 : Gain  Gain=1/den5(1)
  Delay{1,3..5} (4 alike) : Delay  DelayLength=1  SampleTime=Ts
  Klim : Gain  Gain=Klim
  Sum : Sum  Inputs=|+-
  Sum3 : Sum  Inputs=|+-
  Sum4 : Sum  Inputs=|++
  Sum5 : Sum  Inputs=+-|
  a0 : Gain  Gain=num5(1)
  a1 : Gain  Gain=num5(2)
  b1 : Gain  Gain=den5(2)
  b2 : Gain  Gain=den5(3)
  Out : Outport
  wires:
  Delay3/1 -> a1/1  "e(n-1)"
  Delay5/1 -> b2/1  "y(n-2)"
  1/b0/1 -> Out/1, Delay4/1  "y(n)"
  Sum3/1 -> Sum4/1
  Sum4/1 -> 1/b0/1
  b2/1 -> Sum5/2
  Sum5/1 -> Sum4/2
  b1/1 -> Sum5/1
  Delay4/1 -> Delay5/1, b1/1  "y(n-1)"
  a0/1 -> Sum3/1
  a1/1 -> Sum3/2
  Delay1/1 -> Klim/1
  Klim/1 -> Sum/2
  Anti-Windup/1 -> Delay1/1
  Sum/1 -> a0/1, Delay3/1  "e(n)"
  In/1 -> Sum/1

== system TTypeInverter_R2022a/Phase 2/Controllers/Current Controller/Impulse Invariant PR - HC7 ==
  In : Inport
  Anti-Windup : Inport  Port=2
  1/b0 : Gain  Gain=1/den7(1)
  Delay{1,3..5} (4 alike) : Delay  DelayLength=1  SampleTime=Ts
  Klim : Gain  Gain=Klim
  Sum : Sum  Inputs=|+-
  Sum3 : Sum  Inputs=|+-
  Sum4 : Sum  Inputs=|++
  Sum5 : Sum  Inputs=+-|
  a0 : Gain  Gain=num7(1)
  a1 : Gain  Gain=num7(2)
  b1 : Gain  Gain=den7(2)
  b2 : Gain  Gain=den7(3)
  Out : Outport
  wires:
  Delay3/1 -> a1/1  "e(n-1)"
  Delay5/1 -> b2/1  "y(n-2)"
  1/b0/1 -> Out/1, Delay4/1  "y(n)"
  Sum3/1 -> Sum4/1
  Sum4/1 -> 1/b0/1
  b2/1 -> Sum5/2
  Sum5/1 -> Sum4/2
  b1/1 -> Sum5/1
  Delay4/1 -> Delay5/1, b1/1  "y(n-1)"
  a0/1 -> Sum3/1
  a1/1 -> Sum3/2
  Klim/1 -> Sum/2
  Anti-Windup/1 -> Delay1/1
  Delay1/1 -> Klim/1
  Sum/1 -> a0/1, Delay3/1  "e(n)"
  In/1 -> Sum/1

== system TTypeInverter_R2022a/Phase 2/Controllers/Current Controller/Lead-Lag ==
  In : Inport
  Delay : Delay  DelayLength=1  SampleTime=Ts
  Delay1 : Delay  DelayLength=1  SampleTime=Ts
  Gain : Gain  Gain=C_c
  Gain1 : Gain
  Sum : Sum  Inputs=|++
  Sum1 : Sum  Inputs=|++
  a0 : Gain  Gain=a0
  a1 : Gain  Gain=a1
  b0 : Gain  Gain=b0
  b1 : Gain  Gain=b1
  Out : Outport
  wires:
  Gain1/1 -> Out/1
  Gain/1 -> Gain1/1
  In/1 -> Delay/1, a0/1  "e(n)"
  a0/1 -> Sum/1
  Delay/1 -> a1/1  "e(n-1)"
  a1/1 -> Sum/2
  Sum/1 -> Sum1/1
  Delay1/1 -> b1/1  "y(n-1)"
  b1/1 -> Sum1/2
  Sum1/1 -> b0/1
  b0/1 -> Delay1/1, Gain/1  "y(n)"

== system TTypeInverter_R2022a/Phase 2/Controllers/Current Controller/PI Controller ==
  In : Inport
  Delay : Delay  DelayLength=1  SampleTime=Ts
  Gain1 : Gain  Gain=Kpc
  Gain2 : Gain  Gain=Ki
  Gain3 : Gain  Gain=Ts
  Sum2 : Sum  Inputs=++|
  Sum3 : Sum  Inputs=|++
  Out : Outport
  wires:
  Gain1/1 -> Sum2/1
  Gain2/1 -> Gain3/1
  Sum3/1 -> Sum2/2, Delay/1
  Gain3/1 -> Sum3/1
  Delay/1 -> Sum3/2
  In/1 -> Gain1/1, Gain2/1
  Sum2/1 -> Out/1

== system TTypeInverter_R2022a/Phase 2/Controllers/Voltage Controller/Fifth Harmonic ==
  In : Inport
  Anti-Windup : Inport  Port=2
  1/b0 : Gain  Gain=1/(KT(3)*KT(3)+2*omega_w(3)*KT(3)+5*5*omega_o*omega_o)
  Delay1 : Delay  DelayLength=1  SampleTime=Ts
  Delay3 : Delay  SampleTime=Ts
  Delay4 : Delay  DelayLength=1  SampleTime=Ts
  Delay5 : Delay  DelayLength=1  SampleTime=Ts
  Klim : Gain  Gain=Klim
  Sum : Sum  Inputs=|+-
  Sum3 : Sum  Inputs=|+-
  Sum4 : Sum  Inputs=|++
  Sum5 : Sum  Inputs=+-|
  a1 : Gain  Gain=2*Kr(3)*KT(3)*omega_w(3)
  b1 : Gain  Gain=2*KT(3)*KT(3)-2*5*5*omega_o*omega_o
  b2 : Gain  Gain=KT(3)*KT(3)+2*omega_w(3)*KT(3)-5*5*omega_o*omega_o
  Out : Outport
  wires:
  Delay3/1 -> Sum3/2  "e(n-2)"
  Delay5/1 -> b2/1  "y(n-2)"
  Klim/1 -> Sum/2
  1/b0/1 -> Out/1, Delay4/1  "y(n)"
  a1/1 -> Sum4/1
  Sum4/1 -> 1/b0/1
  Sum3/1 -> a1/1
  b2/1 -> Sum5/2
  Sum5/1 -> Sum4/2
  Sum/1 -> Sum3/1, Delay3/1  "e(n)"
  b1/1 -> Sum5/1
  Delay4/1 -> Delay5/1, b1/1  "y(n-1)"
  In/1 -> Sum/1
  Delay1/1 -> Klim/1
  Anti-Windup/1 -> Delay1/1

== system TTypeInverter_R2022a/Phase 2/Controllers/Voltage Controller/Fundamental ==
  In : Inport
  Anti-Windup : Inport  Port=2
  1/b0 : Gain  Gain=1/(KT(1)*KT(1)+2*omega_w(1)*KT(1)+omega_o*omega_o)
  Delay1 : Delay  DelayLength=1  SampleTime=Ts
  Delay3 : Delay  SampleTime=Ts
  Delay4 : Delay  DelayLength=1  SampleTime=Ts
  Delay5 : Delay  DelayLength=1  SampleTime=Ts
  Klim : Gain  Gain=Klim
  Sum : Sum  Inputs=|+-
  Sum3 : Sum  Inputs=|+-
  Sum4 : Sum  Inputs=|++
  Sum5 : Sum  Inputs=+-|
  a1 : Gain  Gain=2*Kr(1)*KT(1)*omega_w(1)
  b1 : Gain  Gain=2*KT(1)*KT(1)-2*omega_o*omega_o
  b2 : Gain  Gain=KT(1)*KT(1)+2*omega_w(1)*KT(1)-omega_o*omega_o
  Out : Outport
  wires:
  Delay3/1 -> Sum3/2  "e(n-2)"
  Delay5/1 -> b2/1  "y(n-2)"
  Klim/1 -> Sum/2
  1/b0/1 -> Out/1, Delay4/1  "y(n)"
  a1/1 -> Sum4/1
  Sum4/1 -> 1/b0/1
  Sum3/1 -> a1/1
  b2/1 -> Sum5/2
  Sum5/1 -> Sum4/2
  Sum/1 -> Sum3/1, Delay3/1  "e(n)"
  b1/1 -> Sum5/1
  Delay4/1 -> Delay5/1, b1/1  "y(n-1)"
  In/1 -> Sum/1
  Delay1/1 -> Klim/1
  Anti-Windup/1 -> Delay1/1

== system TTypeInverter_R2022a/Phase 2/Controllers/Voltage Controller/Impulse Invariant PR - Fundamental ==
  e_out : Inport
  Anti-Windup : Inport  Port=2
  1/b0 : Gain  Gain=1/den(1)
  Delay{1,3..5} (4 alike) : Delay  DelayLength=1  SampleTime=Ts
  Klim : Gain  Gain=Klim
  Sum : Sum  Inputs=|+-
  Sum3 : Sum  Inputs=|+-
  Sum4 : Sum  Inputs=|++
  Sum5 : Sum  Inputs=+-|
  a0 : Gain  Gain=num(1)
  a1 : Gain  Gain=num(2)
  b1 : Gain  Gain=den(2)
  b2 : Gain  Gain=den(3)
  Out : Outport
  wires:
  Delay3/1 -> a1/1  "e(n-1)"
  Delay5/1 -> b2/1  "y(n-2)"
  Klim/1 -> Sum/2
  1/b0/1 -> Out/1, Delay4/1  "y(n)"
  Sum3/1 -> Sum4/1
  Sum4/1 -> 1/b0/1
  b2/1 -> Sum5/2
  Sum5/1 -> Sum4/2
  Sum/1 -> a0/1, Delay3/1  "e(n)"
  b1/1 -> Sum5/1
  Delay4/1 -> Delay5/1, b1/1  "y(n-1)"
  e_out/1 -> Sum/1
  Delay1/1 -> Klim/1
  Anti-Windup/1 -> Delay1/1
  a0/1 -> Sum3/1
  a1/1 -> Sum3/2

== system TTypeInverter_R2022a/Phase 2/Controllers/Voltage Controller/Non-prewarped Tustin-based PR ==
  In1 : Inport
  1/(Ts*Ts*omega_0*omega_0+4*Ts*omega_w+4) : Gain  Gain=1/(Ts*Ts*omega_o*omega_o+4*Ts*omega_w(1)+4)
  2*Ts*Ts*omega_0*omega_0 : Gain  Gain=2*Ts*Ts*omega_o*omega_o-8
  4*Ts*omega_w : Gain  Gain=4*Ts*omega_w(1)
  4*Ts*omega_w! : Gain  Gain=4*Ts*omega_w(1)
  Add1 : Sum
  Delay3 : Delay  SampleTime=Ts
  Delay4 : Delay  DelayLength=1  SampleTime=Ts
  Delay5 : Delay  DelayLength=1  SampleTime=Ts
  Multiply2 : Gain  Gain=Kp
  Multiply3 : Gain  Gain=Kr(1)
  Saturation : Saturate  UpperLimit=pr_sat_val  LowerLimit=-pr_sat_val
  Sum3 : Sum  Inputs=|+-
  Sum4 : Sum  Inputs=|+-
  Sum5 : Sum  Inputs=++|
  Ts*Ts*omega_0*omega_0-4*Ts*omega_w : Gain  Gain=Ts*Ts*omega_o*omega_o-4*Ts*omega_w(1)+4
  Out1 : Outport
  wires:
  Multiply2/1 -> Add1/1
  Delay4/1 -> Delay5/1, 2*Ts*Ts*omega_0*omega_0/1
  Delay5/1 -> Ts*Ts*omega_0*omega_0-4*Ts*omega_w/1
  Multiply3/1 -> Delay3/1, 4*Ts*omega_w/1
  Delay3/1 -> 4*Ts*omega_w!/1
  Sum3/1 -> Sum4/1
  In1/1 -> Multiply3/1, Multiply2/1
  4*Ts*omega_w/1 -> Sum3/1
  Saturation/1 -> Out1/1
  Ts*Ts*omega_0*omega_0-4*Ts*omega_w/1 -> Sum5/2
  4*Ts*omega_w!/1 -> Sum3/2
  Sum5/1 -> Sum4/2
  Sum4/1 -> 1/(Ts*Ts*omega_0*omega_0+4*Ts*omega_w+4)/1
  Add1/1 -> Saturation/1
  1/(Ts*Ts*omega_0*omega_0+4*Ts*omega_w+4)/1 -> Add1/2, Delay4/1
  2*Ts*Ts*omega_0*omega_0/1 -> Sum5/1

== system TTypeInverter_R2022a/Phase 2/Controllers/Voltage Controller/Seventh Harmonic ==
  In : Inport
  Anti-Windup : Inport  Port=2
  1/b0 : Gain  Gain=1/(KT(4)*KT(4)+2*omega_w(4)*KT(4)+7*omega_o*omega_o)
  Delay1 : Delay  DelayLength=1  SampleTime=Ts
  Delay3 : Delay  SampleTime=Ts
  Delay4 : Delay  DelayLength=1  SampleTime=Ts
  Delay5 : Delay  DelayLength=1  SampleTime=Ts
  Klim : Gain  Gain=Klim
  Sum : Sum  Inputs=|+-
  Sum3 : Sum  Inputs=|+-
  Sum4 : Sum  Inputs=|++
  Sum5 : Sum  Inputs=+-|
  a1 : Gain  Gain=2*Kr(4)*KT(4)*omega_w(4)
  b1 : Gain  Gain=2*KT(4)*KT(4)-2*7*omega_o*omega_o
  b2 : Gain  Gain=KT(4)*KT(4)+2*omega_w(4)*KT(4)-7*omega_o*omega_o
  Out : Outport
  wires:
  Delay3/1 -> Sum3/2  "e(n-2)"
  Delay5/1 -> b2/1  "y(n-2)"
  Klim/1 -> Sum/2
  1/b0/1 -> Out/1, Delay4/1  "y(n)"
  a1/1 -> Sum4/1
  Sum4/1 -> 1/b0/1
  Sum3/1 -> a1/1
  b2/1 -> Sum5/2
  Sum5/1 -> Sum4/2
  Sum/1 -> Sum3/1, Delay3/1  "e(n)"
  b1/1 -> Sum5/1
  Delay4/1 -> Delay5/1, b1/1  "y(n-1)"
  In/1 -> Sum/1
  Delay1/1 -> Klim/1
  Anti-Windup/1 -> Delay1/1

== system TTypeInverter_R2022a/Phase 2/Controllers/Voltage Controller/Third Harmonic ==
  In : Inport
  Anti-Windup : Inport  Port=2
  1/b0 : Gain  Gain=1/(KT(2)*KT(2)+2*omega_w(2)*KT(2)+3*3*omega_o*omega_o)
  Delay1 : Delay  DelayLength=1  SampleTime=Ts
  Delay3 : Delay  SampleTime=Ts
  Delay4 : Delay  DelayLength=1  SampleTime=Ts
  Delay5 : Delay  DelayLength=1  SampleTime=Ts
  Klim : Gain  Gain=Klim
  Sum : Sum  Inputs=|+-
  Sum3 : Sum  Inputs=|+-
  Sum4 : Sum  Inputs=|++
  Sum5 : Sum  Inputs=+-|
  a1 : Gain  Gain=2*Kr(2)*KT(2)*omega_w(2)
  b1 : Gain  Gain=2*KT(2)*KT(2)-2*3*3*omega_o*omega_o
  b2 : Gain  Gain=KT(2)*KT(2)+2*omega_w(2)*KT(2)-3*3*omega_o*omega_o
  Out : Outport
  wires:
  Delay3/1 -> Sum3/2  "e(n-2)"
  Delay5/1 -> b2/1  "y(n-2)"
  Klim/1 -> Sum/2
  1/b0/1 -> Out/1, Delay4/1  "y(n)"
  a1/1 -> Sum4/1
  Sum4/1 -> 1/b0/1
  Sum3/1 -> a1/1
  b2/1 -> Sum5/2
  Sum5/1 -> Sum4/2
  Sum/1 -> Sum3/1, Delay3/1  "e(n)"
  b1/1 -> Sum5/1
  Delay4/1 -> Delay5/1, b1/1  "y(n-1)"
  In/1 -> Sum/1
  Delay1/1 -> Klim/1
  Anti-Windup/1 -> Delay1/1

== system TTypeInverter_R2022a/Phase 3/Controllers/Current Controller/Impulse Invariant PR - HC15 ==
  e_out : Inport
  Anti-Windup : Inport  Port=2
  1/b0 : Gain  Gain=1/den15(1)
  Delay{1,3..5} (4 alike) : Delay  DelayLength=1  SampleTime=Ts
  Klim : Gain  Gain=Klim
  Sum : Sum  Inputs=|+-
  Sum3 : Sum  Inputs=|+-
  Sum4 : Sum  Inputs=|++
  Sum5 : Sum  Inputs=+-|
  a0 : Gain  Gain=num15(1)
  a1 : Gain  Gain=num15(2)
  b1 : Gain  Gain=den15(2)
  b2 : Gain  Gain=den15(3)
  Out : Outport
  wires:
  Delay3/1 -> a1/1  "e(n-1)"
  Delay5/1 -> b2/1  "y(n-2)"
  1/b0/1 -> Out/1, Delay4/1  "y(n)"
  Sum3/1 -> Sum4/1
  Sum4/1 -> 1/b0/1
  b2/1 -> Sum5/2
  Sum5/1 -> Sum4/2
  b1/1 -> Sum5/1
  Delay4/1 -> Delay5/1, b1/1  "y(n-1)"
  a0/1 -> Sum3/1
  a1/1 -> Sum3/2
  Klim/1 -> Sum/2
  Anti-Windup/1 -> Delay1/1
  Delay1/1 -> Klim/1
  Sum/1 -> a0/1, Delay3/1  "e(n)"
  e_out/1 -> Sum/1

== system TTypeInverter_R2022a/Phase 3/Controllers/Current Controller/Impulse Invariant PR - HC21 ==
  e_out : Inport
  Anti-Windup : Inport  Port=2
  1/b0 : Gain  Gain=1/den21(1)
  Delay{1,3..5} (4 alike) : Delay  DelayLength=1  SampleTime=Ts
  Klim : Gain  Gain=Klim
  Sum : Sum  Inputs=|+-
  Sum3 : Sum  Inputs=|+-
  Sum4 : Sum  Inputs=|++
  Sum5 : Sum  Inputs=+-|
  a0 : Gain  Gain=num21(1)
  a1 : Gain  Gain=num21(2)
  b1 : Gain  Gain=den21(2)
  b2 : Gain  Gain=den21(3)
  Out : Outport
  wires:
  Delay3/1 -> a1/1  "e(n-1)"
  Delay5/1 -> b2/1  "y(n-2)"
  1/b0/1 -> Out/1, Delay4/1  "y(n)"
  Sum3/1 -> Sum4/1
  Sum4/1 -> 1/b0/1
  b2/1 -> Sum5/2
  Sum5/1 -> Sum4/2
  b1/1 -> Sum5/1
  Delay4/1 -> Delay5/1, b1/1  "y(n-1)"
  a0/1 -> Sum3/1
  a1/1 -> Sum3/2
  Klim/1 -> Sum/2
  Anti-Windup/1 -> Delay1/1
  Delay1/1 -> Klim/1
  Sum/1 -> a0/1, Delay3/1  "e(n)"
  e_out/1 -> Sum/1

== system TTypeInverter_R2022a/Phase 3/Controllers/Current Controller/Impulse Invariant PR - HC5 ==
  In : Inport
  Anti-Windup : Inport  Port=2
  1/b0 : Gain  Gain=1/den5(1)
  Delay{1,3..5} (4 alike) : Delay  DelayLength=1  SampleTime=Ts
  Klim : Gain  Gain=Klim
  Sum : Sum  Inputs=|+-
  Sum3 : Sum  Inputs=|+-
  Sum4 : Sum  Inputs=|++
  Sum5 : Sum  Inputs=+-|
  a0 : Gain  Gain=num5(1)
  a1 : Gain  Gain=num5(2)
  b1 : Gain  Gain=den5(2)
  b2 : Gain  Gain=den5(3)
  Out : Outport
  wires:
  Delay3/1 -> a1/1  "e(n-1)"
  Delay5/1 -> b2/1  "y(n-2)"
  1/b0/1 -> Out/1, Delay4/1  "y(n)"
  Sum3/1 -> Sum4/1
  Sum4/1 -> 1/b0/1
  b2/1 -> Sum5/2
  Sum5/1 -> Sum4/2
  b1/1 -> Sum5/1
  Delay4/1 -> Delay5/1, b1/1  "y(n-1)"
  a0/1 -> Sum3/1
  a1/1 -> Sum3/2
  Delay1/1 -> Klim/1
  Klim/1 -> Sum/2
  Anti-Windup/1 -> Delay1/1
  Sum/1 -> a0/1, Delay3/1  "e(n)"
  In/1 -> Sum/1

== system TTypeInverter_R2022a/Phase 3/Controllers/Current Controller/Impulse Invariant PR - HC7 ==
  In : Inport
  Anti-Windup : Inport  Port=2
  1/b0 : Gain  Gain=1/den7(1)
  Delay{1,3..5} (4 alike) : Delay  DelayLength=1  SampleTime=Ts
  Klim : Gain  Gain=Klim
  Sum : Sum  Inputs=|+-
  Sum3 : Sum  Inputs=|+-
  Sum4 : Sum  Inputs=|++
  Sum5 : Sum  Inputs=+-|
  a0 : Gain  Gain=num7(1)
  a1 : Gain  Gain=num7(2)
  b1 : Gain  Gain=den7(2)
  b2 : Gain  Gain=den7(3)
  Out : Outport
  wires:
  Delay3/1 -> a1/1  "e(n-1)"
  Delay5/1 -> b2/1  "y(n-2)"
  1/b0/1 -> Out/1, Delay4/1  "y(n)"
  Sum3/1 -> Sum4/1
  Sum4/1 -> 1/b0/1
  b2/1 -> Sum5/2
  Sum5/1 -> Sum4/2
  b1/1 -> Sum5/1
  Delay4/1 -> Delay5/1, b1/1  "y(n-1)"
  a0/1 -> Sum3/1
  a1/1 -> Sum3/2
  Klim/1 -> Sum/2
  Anti-Windup/1 -> Delay1/1
  Delay1/1 -> Klim/1
  Sum/1 -> a0/1, Delay3/1  "e(n)"
  In/1 -> Sum/1

== system TTypeInverter_R2022a/Phase 3/Controllers/Current Controller/Lead-Lag ==
  In : Inport
  Delay : Delay  DelayLength=1  SampleTime=Ts
  Delay1 : Delay  DelayLength=1  SampleTime=Ts
  Gain : Gain  Gain=C_c
  Gain1 : Gain
  Sum : Sum  Inputs=|++
  Sum1 : Sum  Inputs=|++
  a0 : Gain  Gain=a0
  a1 : Gain  Gain=a1
  b0 : Gain  Gain=b0
  b1 : Gain  Gain=b1
  Out : Outport
  wires:
  Gain1/1 -> Out/1
  Gain/1 -> Gain1/1
  In/1 -> Delay/1, a0/1  "e(n)"
  a0/1 -> Sum/1
  Delay/1 -> a1/1  "e(n-1)"
  a1/1 -> Sum/2
  Sum/1 -> Sum1/1
  Delay1/1 -> b1/1  "y(n-1)"
  b1/1 -> Sum1/2
  Sum1/1 -> b0/1
  b0/1 -> Delay1/1, Gain/1  "y(n)"

== system TTypeInverter_R2022a/Phase 3/Controllers/Current Controller/PI Controller ==
  In : Inport
  Delay : Delay  DelayLength=1  SampleTime=Ts
  Gain1 : Gain  Gain=Kpc
  Gain2 : Gain  Gain=Ki
  Gain3 : Gain  Gain=Ts
  Sum2 : Sum  Inputs=++|
  Sum3 : Sum  Inputs=|++
  Out : Outport
  wires:
  Gain1/1 -> Sum2/1
  Gain2/1 -> Gain3/1
  Sum3/1 -> Sum2/2, Delay/1
  Gain3/1 -> Sum3/1
  Delay/1 -> Sum3/2
  In/1 -> Gain1/1, Gain2/1
  Sum2/1 -> Out/1

== system TTypeInverter_R2022a/Phase 3/Controllers/Voltage Controller/Fifth Harmonic ==
  In : Inport
  Anti-Windup : Inport  Port=2
  1/b0 : Gain  Gain=1/(KT(3)*KT(3)+2*omega_w(3)*KT(3)+5*5*omega_o*omega_o)
  Delay1 : Delay  DelayLength=1  SampleTime=Ts
  Delay3 : Delay  SampleTime=Ts
  Delay4 : Delay  DelayLength=1  SampleTime=Ts
  Delay5 : Delay  DelayLength=1  SampleTime=Ts
  Klim : Gain  Gain=Klim
  Sum : Sum  Inputs=|+-
  Sum3 : Sum  Inputs=|+-
  Sum4 : Sum  Inputs=|++
  Sum5 : Sum  Inputs=+-|
  a1 : Gain  Gain=2*Kr(3)*KT(3)*omega_w(3)
  b1 : Gain  Gain=2*KT(3)*KT(3)-2*5*5*omega_o*omega_o
  b2 : Gain  Gain=KT(3)*KT(3)+2*omega_w(3)*KT(3)-5*5*omega_o*omega_o
  Out : Outport
  wires:
  Delay3/1 -> Sum3/2  "e(n-2)"
  Delay5/1 -> b2/1  "y(n-2)"
  Klim/1 -> Sum/2
  1/b0/1 -> Out/1, Delay4/1  "y(n)"
  a1/1 -> Sum4/1
  Sum4/1 -> 1/b0/1
  Sum3/1 -> a1/1
  b2/1 -> Sum5/2
  Sum5/1 -> Sum4/2
  Sum/1 -> Sum3/1, Delay3/1  "e(n)"
  b1/1 -> Sum5/1
  Delay4/1 -> Delay5/1, b1/1  "y(n-1)"
  In/1 -> Sum/1
  Delay1/1 -> Klim/1
  Anti-Windup/1 -> Delay1/1

== system TTypeInverter_R2022a/Phase 3/Controllers/Voltage Controller/Fundamental ==
  In : Inport
  Anti-Windup : Inport  Port=2
  1/b0 : Gain  Gain=1/(KT(1)*KT(1)+2*omega_w(1)*KT(1)+omega_o*omega_o)
  Delay1 : Delay  DelayLength=1  SampleTime=Ts
  Delay3 : Delay  SampleTime=Ts
  Delay4 : Delay  DelayLength=1  SampleTime=Ts
  Delay5 : Delay  DelayLength=1  SampleTime=Ts
  Klim : Gain  Gain=Klim
  Sum : Sum  Inputs=|+-
  Sum3 : Sum  Inputs=|+-
  Sum4 : Sum  Inputs=|++
  Sum5 : Sum  Inputs=+-|
  a1 : Gain  Gain=2*Kr(1)*KT(1)*omega_w(1)
  b1 : Gain  Gain=2*KT(1)*KT(1)-2*omega_o*omega_o
  b2 : Gain  Gain=KT(1)*KT(1)+2*omega_w(1)*KT(1)-omega_o*omega_o
  Out : Outport
  wires:
  Delay3/1 -> Sum3/2  "e(n-2)"
  Delay5/1 -> b2/1  "y(n-2)"
  Klim/1 -> Sum/2
  1/b0/1 -> Out/1, Delay4/1  "y(n)"
  a1/1 -> Sum4/1
  Sum4/1 -> 1/b0/1
  Sum3/1 -> a1/1
  b2/1 -> Sum5/2
  Sum5/1 -> Sum4/2
  Sum/1 -> Sum3/1, Delay3/1  "e(n)"
  b1/1 -> Sum5/1
  Delay4/1 -> Delay5/1, b1/1  "y(n-1)"
  In/1 -> Sum/1
  Delay1/1 -> Klim/1
  Anti-Windup/1 -> Delay1/1

== system TTypeInverter_R2022a/Phase 3/Controllers/Voltage Controller/Impulse Invariant PR - Fundamental ==
  e_out : Inport
  Anti-Windup : Inport  Port=2
  1/b0 : Gain  Gain=1/den(1)
  Delay{1,3..5} (4 alike) : Delay  DelayLength=1  SampleTime=Ts
  Klim : Gain  Gain=Klim
  Sum : Sum  Inputs=|+-
  Sum3 : Sum  Inputs=|+-
  Sum4 : Sum  Inputs=|++
  Sum5 : Sum  Inputs=+-|
  a0 : Gain  Gain=num(1)
  a1 : Gain  Gain=num(2)
  b1 : Gain  Gain=den(2)
  b2 : Gain  Gain=den(3)
  Out : Outport
  wires:
  Delay3/1 -> a1/1  "e(n-1)"
  Delay5/1 -> b2/1  "y(n-2)"
  Klim/1 -> Sum/2
  1/b0/1 -> Out/1, Delay4/1  "y(n)"
  Sum3/1 -> Sum4/1
  Sum4/1 -> 1/b0/1
  b2/1 -> Sum5/2
  Sum5/1 -> Sum4/2
  Sum/1 -> a0/1, Delay3/1  "e(n)"
  b1/1 -> Sum5/1
  Delay4/1 -> Delay5/1, b1/1  "y(n-1)"
  e_out/1 -> Sum/1
  Delay1/1 -> Klim/1
  Anti-Windup/1 -> Delay1/1
  a0/1 -> Sum3/1
  a1/1 -> Sum3/2

== system TTypeInverter_R2022a/Phase 3/Controllers/Voltage Controller/Non-prewarped Tustin-based PR ==
  In1 : Inport
  1/(Ts*Ts*omega_0*omega_0+4*Ts*omega_w+4) : Gain  Gain=1/(Ts*Ts*omega_o*omega_o+4*Ts*omega_w(1)+4)
  2*Ts*Ts*omega_0*omega_0 : Gain  Gain=2*Ts*Ts*omega_o*omega_o-8
  4*Ts*omega_w : Gain  Gain=4*Ts*omega_w(1)
  4*Ts*omega_w! : Gain  Gain=4*Ts*omega_w(1)
  Add1 : Sum
  Delay3 : Delay  SampleTime=Ts
  Delay4 : Delay  DelayLength=1  SampleTime=Ts
  Delay5 : Delay  DelayLength=1  SampleTime=Ts
  Multiply2 : Gain  Gain=Kp
  Multiply3 : Gain  Gain=Kr(1)
  Saturation : Saturate  UpperLimit=pr_sat_val  LowerLimit=-pr_sat_val
  Sum3 : Sum  Inputs=|+-
  Sum4 : Sum  Inputs=|+-
  Sum5 : Sum  Inputs=++|
  Ts*Ts*omega_0*omega_0-4*Ts*omega_w : Gain  Gain=Ts*Ts*omega_o*omega_o-4*Ts*omega_w(1)+4
  Out1 : Outport
  wires:
  Multiply2/1 -> Add1/1
  Delay4/1 -> Delay5/1, 2*Ts*Ts*omega_0*omega_0/1
  Delay5/1 -> Ts*Ts*omega_0*omega_0-4*Ts*omega_w/1
  Multiply3/1 -> Delay3/1, 4*Ts*omega_w/1
  Delay3/1 -> 4*Ts*omega_w!/1
  Sum3/1 -> Sum4/1
  In1/1 -> Multiply3/1, Multiply2/1
  4*Ts*omega_w/1 -> Sum3/1
  Saturation/1 -> Out1/1
  Ts*Ts*omega_0*omega_0-4*Ts*omega_w/1 -> Sum5/2
  4*Ts*omega_w!/1 -> Sum3/2
  Sum5/1 -> Sum4/2
  Sum4/1 -> 1/(Ts*Ts*omega_0*omega_0+4*Ts*omega_w+4)/1
  Add1/1 -> Saturation/1
  1/(Ts*Ts*omega_0*omega_0+4*Ts*omega_w+4)/1 -> Add1/2, Delay4/1
  2*Ts*Ts*omega_0*omega_0/1 -> Sum5/1

== system TTypeInverter_R2022a/Phase 3/Controllers/Voltage Controller/Seventh Harmonic ==
  In : Inport
  Anti-Windup : Inport  Port=2
  1/b0 : Gain  Gain=1/(KT(4)*KT(4)+2*omega_w(4)*KT(4)+7*omega_o*omega_o)
  Delay1 : Delay  DelayLength=1  SampleTime=Ts
  Delay3 : Delay  SampleTime=Ts
  Delay4 : Delay  DelayLength=1  SampleTime=Ts
  Delay5 : Delay  DelayLength=1  SampleTime=Ts
  Klim : Gain  Gain=Klim
  Sum : Sum  Inputs=|+-
  Sum3 : Sum  Inputs=|+-
  Sum4 : Sum  Inputs=|++
  Sum5 : Sum  Inputs=+-|
  a1 : Gain  Gain=2*Kr(4)*KT(4)*omega_w(4)
  b1 : Gain  Gain=2*KT(4)*KT(4)-2*7*omega_o*omega_o
  b2 : Gain  Gain=KT(4)*KT(4)+2*omega_w(4)*KT(4)-7*omega_o*omega_o
  Out : Outport
  wires:
  Delay3/1 -> Sum3/2  "e(n-2)"
  Delay5/1 -> b2/1  "y(n-2)"
  Klim/1 -> Sum/2
  1/b0/1 -> Out/1, Delay4/1  "y(n)"
  a1/1 -> Sum4/1
  Sum4/1 -> 1/b0/1
  Sum3/1 -> a1/1
  b2/1 -> Sum5/2
  Sum5/1 -> Sum4/2
  Sum/1 -> Sum3/1, Delay3/1  "e(n)"
  b1/1 -> Sum5/1
  Delay4/1 -> Delay5/1, b1/1  "y(n-1)"
  In/1 -> Sum/1
  Delay1/1 -> Klim/1
  Anti-Windup/1 -> Delay1/1
